simulink model "sl_subsys_for1"  (Simulink 7.6)
settings: Solver=FixedStepDiscrete  StartTime=0.0  StopTime=10.0  FixedStep=1  RelTol=1e-3
Description:
  | For-subsystem that is used to compute the sum of the numbers between 1 and N
settings Model: Creator=The MathWorks Inc.  CovMetricSettings=d  ExtModeAutoUpdateStatusClock=off
settings OptimizationCC: BlockReduction=off  BooleanDataType=off  InlineInvariantSignals=on  InitFltsAndDblsToZero=on
settings DebuggingCC: SaveWithParameterizedLinksMsg=none  SignalResolutionControl=TryResolveAllWithWarning  SolverPrmCheckMsg=none  MultiTaskDSMMsg=warning  MultiTaskCondExecSysMsg=none
settings HardwareCC: TargetUnknown=on
settings RTWCC: IncludeERTFirstTime=on
settings CodeAppCC: CustomSymbolStrFcn=$F$N$M
settings GRTTargetCC: TargetFcnLib=ansi_tfl_tmw.mat

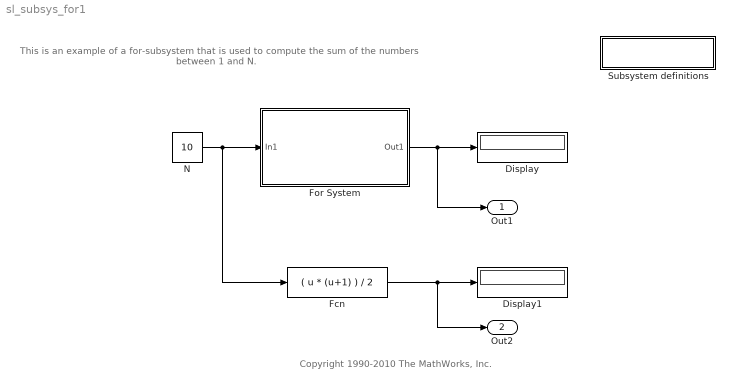
== system sl_subsys_for1 ==
  note: This is an example of a for-subsystem that is used
      | to compute the sum of the numbers between 1 and N.
  note: Copyright 1990-2010 The MathWorks, Inc.
  " Subsystem definitions" : Subsystem
      settings: OpenFcn=helpview([matlabroot,'/toolbox/simulink/simdemos/simfeatures/html/sl_subsys_definitions.html']);
      mask Display: disp('Subsystem\ndefinitions')
  Display : Display
  Display1 : Display
  Fcn : Fcn  Expr=( u * (u+1) ) / 2
  For System : Subsystem  TreatAsAtomicUnit=on
  N : Constant  Value=10
  Out1 : Outport
  Out2 : Outport  Port=2
  wires:
  N/1 -> For System/1(In1), Fcn/1
  For System/1(Out1) -> Display/1, Out1/1
  Fcn/1 -> Display1/1, Out2/1

== system sl_subsys_for1/ Subsystem definitions ==

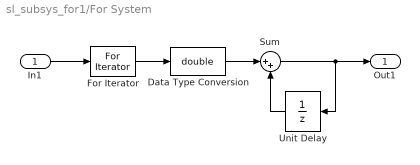
== system sl_subsys_for1/For System ==
  In1 : Inport
  Data Type Conversion : DataTypeConversion  OutDataTypeStr=double  SaturateOnIntegerOverflow=on  RndMeth=Zero
  For Iterator : ForIterator  ResetStates=reset  IterationSource=external
  Sum : Sum  Inputs=|++  SaturateOnIntegerOverflow=on  InputSameDT=on  OutDataTypeStr=Inherit: Same as first input
  Unit Delay : UnitDelay  SampleTime=-1
  Out1 : Outport
  wires:
  Sum/1 -> Unit Delay/1, Out1/1
  For Iterator/1 -> Data Type Conversion/1
  In1/1 -> For Iterator/1
  Unit Delay/1 -> Sum/2
  Data Type Conversion/1 -> Sum/1
